simulink model "speed_regulator_r2022b_empty"  (R2022b)
settings: Solver=ode4  StartTime=0.0  StopTime=Inf  FixedStep=0.5  RelTol=1e-3  AbsTol=1e-6
settings Model: Creator=dmedonza  LastModifiedBy=fabriziosossan
settings SolverCC: AutoScaleAbsTol=off  AlgebraicLoopSolver=TrustRegion
settings DataIOCC: LimitDataPoints=on  SaveFormat=Array  SignalLoggingSaveFormat=ModelDataLogs  SaveOutput=off  SignalLogging=off  SaveTime=off  ReturnWorkspaceOutputs=off
settings OptimizationCC: BooleanDataType=off  ExpressionDepthLimit=2147483647  LifeSpan=inf
settings DebuggingCC: SaveWithParameterizedLinksMsg=none  UnderspecifiedInitializationDetection=Classic  MergeDetectMultiDrivingBlocksExec=none  SignalResolutionControl=TryResolveAllWithWarning  MultiTaskDSMMsg=warning  MultiTaskCondExecSysMsg=none  FcnCallInpInsideContextMsg=warning  UnconnectedInputMsg=warning  UnconnectedOutputMsg=warning  UnconnectedLineMsg=warning  StateNameClashWarn=warning  SFUnexpectedBacktrackingDiag=warning  SFNoUnconditionalDefaultTransitionDiag=warning  SFExecutionAtInitializationDiag=none  SFMachineParentedDataDiag=warning  ArithmeticOperatorsInVariantConditions=warning
settings HardwareCC: ProdBitPerPointer=32  ProdBitPerSizeT=32  ProdBitPerPtrDiffT=32  ProdLargestAtomicFloat=None  ProdIntDivRoundTo=Undefined  ProdEndianess=Unspecified  ProdWordSize=32  ProdHWDeviceType=32-bit Generic  TargetUnknown=on
settings ModelReferenceCC: PropagateSignalLabelsOutOfModel=off
settings SFSimCC: SimUseLocalCustomCode=off  CustomCodeUndefinedFunction=UseInterfaceOnly
settings RTWCC: TemplateMakefile=grt_vc.tmf  RTWUseLocalCustomCode=off
settings CodeAppCC: StateflowObjectComments=on
settings GRTTargetCC: TargetLangStandard=C89/C90 (ANSI)  CombineOutputUpdateFcns=off  GRTInterface=on
settings ConfigComp: CovMetricSettings=dw  CovSaveCumulativeToWorkspaceVar=on  CovSaveSingleToWorkspaceVar=on  CovExternalEMLEnable=off

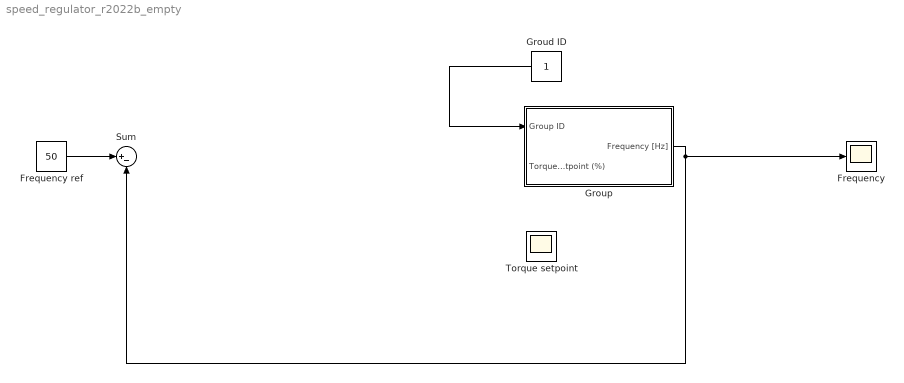
== system speed_regulator_r2022b_empty ==
  Frequency : Scope
  Frequency ref : Constant  Value=50
  Groud ID : Constant
  Group : Subsystem
  Sum : Sum  Inputs=|+-
  Torque setpoint : Scope
  wires:
  Groud ID/1 -> Group/1(Group ID)
  Frequency ref/1 -> Sum/1
  Group/1(Frequency [Hz]) -> Frequency/1, Sum/2

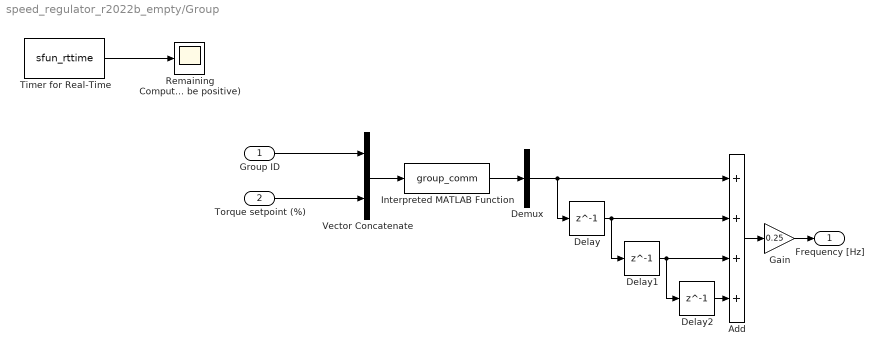
== system speed_regulator_r2022b_empty/Group ==
  Group ID : Inport
  Torque setpoint (%) : Inport  Port=2
  Add : Sum  Inputs=++++
  Delay : Delay  DelayLength=1  InitialCondition=0
  Delay1 : Delay  DelayLength=1  InitialCondition=0
  Delay2 : Delay  DelayLength=1  InitialCondition=0
  Demux : Demux  Outputs=1
  Gain : Gain  Gain=0.25
  Interpreted MATLAB Function : MATLABFcn  MATLABFcn=group_comm
  Remaining Computation Time (must be positive) : Scope
  Timer for Real-Time : S-Function  FunctionName=sfun_rttime  Parameters=1  SFunctionDeploymentMode=off  EnableBusSupport=off
  Vector Concatenate : Concatenate
  Frequency [Hz] : Outport
  wires:
  Torque setpoint (%)/1 -> Vector Concatenate/2
  Group ID/1 -> Vector Concatenate/1
  Vector Concatenate/1 -> Interpreted MATLAB Function/1
  Interpreted MATLAB Function/1 -> Demux/1
  Timer for Real-Time/1 -> Remaining Computation Time (must be positive)/1
  Demux/1 -> Delay/1, Add/1
  Delay/1 -> Add/2, Delay1/1
  Delay1/1 -> Delay2/1, Add/3
  Delay2/1 -> Add/4
  Gain/1 -> Frequency [Hz]/1
  Add/1 -> Gain/1
